simulink model "ARC_DTm"  (R2025b)
settings: Solver=FixedStepAuto  StartTime=0.0  StopTime=10080  FixedStep=1  RelTol=1e-3
PreLoadFcn:
  | %For Preload, set the working path
  | modelFolder = fileparts(which(bdroot));
  | addpath(genpath(modelFolder));
StartFcn:
  | tic
StopFcn:
  | fprintf("Sim Time: %.02f min", toc/60)
values from neighbouring files (symbols this model uses):
  batteryScenario = p.batteryScenario    [RUNSIM_ParameterSweep.m]    (also in _RUNSIM_ParameterSweep.m)
  Electricity_SalePriceModifier = 50/100    (= 0.5)    [RUNSIM_ParameterSweep.m]    (also in _RUNSIM_ParameterSweep.m)
  LUT = LUT_load.gamLUT    [RUNSIM_ParameterSweep.m]    (also in _RUNSIM_ParameterSweep.m)
  minimum_UF_system_flow = 5833    [RUNSIM_ParameterSweep.m]    (also in _RUNSIM_ParameterSweep.m)
  PROS1_recoveryrate = 61    [RUNSIM_ParameterSweep.m]    (also in _RUNSIM_ParameterSweep.m)
  PROS2_recoveryrate = 62    [RUNSIM_ParameterSweep.m]    (also in _RUNSIM_ParameterSweep.m)
  ROstabilization_time = p.ROstabilization_time    [RUNSIM_ParameterSweep.m]    (also in _RUNSIM_ParameterSweep.m)
  solarModifier = maximum_solar_generation / 300    [RUNSIM_ParameterSweep.m]    (also in _RUNSIM_ParameterSweep.m)
  TSRO_recoveryrate = 51    [RUNSIM_ParameterSweep.m]    (also in _RUNSIM_ParameterSweep.m)
  UF_RecoveryRate = 96    [RUNSIM_ParameterSweep.m]    (also in _RUNSIM_ParameterSweep.m)
undefined symbols (not defined in the file or in its folder): A_PROS1, A_PROS2, A_TSRO, B_PROS1, B_PROS2, B_TSRO, BW_Max_Time, BW_Max_Vol_gal, CEB_Max_Time, CEB_Max_Vol_gal, CIP_Max_Time, E, FF, h, L, w
libraries: simulink x40
(part 3 of 11)

== system ARC_DTm/Plant_LocalLoad_FMU ==
  note: Time-of-Use Scenarios are defined in the input spreadsheet 'OperationalScenarios.xlsx'. This subsystem allows a toggling of scenarios through modifying the TOU_Rate_Scenario constant block in the MATLAB editor.
  note: Net Power
  note: PRO_1
  note: Import UF Power
  note: PRO_2
  note: PRO_3
  note: PRO_4
  note: This subsystem utilizes the FMU and battery logic developed by the Electric Power Research Institute (EPRI) to simulate the potential impact of an on-site battery under different charge and discharge control scenarios.
  Abs : Abs  SaturateOnIntegerOverflow=off
  Abs1 : Abs  SaturateOnIntegerOverflow=off
  Add : Sum
  Add1 : Sum  Inputs=++++
  Add2 : Sum  Inputs=++++++++
  Add3 : Sum  Inputs=++++
  Battery System : Subsystem
  Bus Creator : BusCreator  Inputs=27
  Constant : Constant  Value=0
  Decarb Off : Constant  Value=0
  Decarbonator Power Demand_kW : Constant  Value=2.5
  Demux : Demux
  Energy Summary : Scope  NumInputPorts=4
      settings: ActiveDisplayYMinimum=-0.12499999999999997  ActiveDisplayYMaximum=1.125  DataLoggingVariableName=ScopeData20
  FMU : FMU  FMUName=HybridPowerControls_EPRI.fmu  FMUDebugLogging=on  FMUMode=CoSimulation  FMUInitializeEnumObject=off  FMUCachedDialogLayout="{\"Geometry\":[0,186,578,484],\"ParameterColumnsWidthConfig\":\"{\\\"columns\\\":[{\\\"name\\\":\\\"Parameter\\\",\\\"width\\\":154},{\\\"name\\\":\\\"Value\\\",\\\"width\\\":59},{\\\"name\\\":\\\"Calculated Value\\\",\\\"width\\\":203},{\\\"name\\\":\\\"Unit\\\",\\\"width\\\":108},{\\\"name\\\":\\\"Description\\\",\\\"width\\\":161}]}\",\"InputColumnsWidthConfig\":\"{\\\"columns\\\":[{\\\"name\\\":\\\"Name\\\",\\\"width\\\":150},{\\\"name\\\":\\\"Visibility\\\",\\\"width\\\":79},{\\\"name\\\":\\\"Start\\\",\\\"width\\\":139},{\\\"name\\\":\\\"Unit\\\",\\\"width\\\":136},{\\\"name\\\":\\\"Type Object\\\",\\\"width\\\":194}]}\",\"OutputColumnsWidthConfig\":\"{\\\"columns\\\":[{\\\"name\\\":\\\"Name\\\",\\\"width\\\":150},{\\\"name\\\":\\\"Visibility\\\",\\\"width\\\":79},{\\\"name\\\":\\\"Start\\\",\\\"width\\\":139},{\\\"name\\\":\\\"Unit\\\",\\\"width\\\":136},{\\\"name\\\":\\\"Type Object\\\",\\\"width\\\":194}]}\"}"  DCDC=struct('P_rat',0,'P_ref',5.0E7,'V_ref',1.0,'capex_ref',1.0,'componentEconomy',struct('annualCapex',0,'capex',0,'cashFlowPerSecond',0,'fixedAnnualOpex',0,'lifetime',0,'summary',struct('capex',0)),'constraint_prim',struct('upperLimitFixed',1.0),'constraint_sec',struct('lowerLimitFixed',-1.0,'upperLimitFixed',1.0),'eta',1.0,'fixedAnnualOpex_ref',1.0,'lifetime',1.0,'pin_prim',struct('v',0),'pin_sec',struct('v',0),'scalingFactor',1.0,'scalingFactor_max',10.0,'scalingFactor_min',0.1,'smoothingPercentage',2.0)  PID_charge=struct('Dzero',struct('k',0.0,'y',0),'FFzero',struct('k',0.0,'y',0),'I',struct('k',0,'y_start',0),'Nd',10.0,'Ni',0.9,'P',struct('k',1.0),'Td',0.1,'Ti',0.025,'addFF',struct('k1',1.0,'k2',0,'u2',0),'addI',struct('k1',1.0,'k2',-1.0,'k3',1.0),'addP',struct('k1',0,'k2',-1.0),'addPID',struct('k1',1.0,'k2',1.0,'k3',1.0,'u2',0),'addSat',struct('k1',1.0,'k2',-1.0),'gainPID',struct('k',0),'gainTrack',struct('k',0),'k',0.16,'kFF',1.0,'wd',0.0,'wp',1.0,'xd_start',0.0,'xi_start',0.0)  PID_discharge=struct('Dzero',struct('k',0.0,'y',0),'FFzero',struct('k',0.0,'y',0),'I',struct('k',0,'y_start',0),'Nd',10.0,'Ni',0.9,'P',struct('k',1.0),'Td',0.1,'Ti',0.025,'addFF',struct('k1',1.0,'k2',0,'u2',0),'addI',struct('k1',1.0,'k2',-1.0,'k3',1.0),'addP',struct('k1',0,'k2',-1.0),'addPID',struct('k1',1.0,'k2',1.0,'k3',1.0,'u2',0),'addSat',struct('k1',1.0,'k2',-1.0),'gainPID',struct('k',0),'gainTrack',struct('k',0),'k',0.16,'kFF',1.0,'wd',0.0,'wp',1.0,'xd_start',0.0,'xi_start',0.0)  P_block_jacobian_check=off  P_block_jacobian_check_tol=1.0E-6  P_block_solver_experimental_mode=int32(0)  P_block_solver_profiling=off  P_cs_experimental_mode=int32(0)  P_cs_profiling=off  P_cs_rel_tol=1.0E-6  P_cs_solver=int32(0)  P_cs_step_size=0.001  P_enforce_bounds=on  P_events_default_tol=1.0E-10  P_events_tol_factor=1.0E-4  P_iteration_variable_scaling=int32(1)  P_log_level=int32(3)  P_log_start_time=-1.0E20  P_log_stop_time=1.0E20  P_mathematical_domain_warnings_limit=int32(-1)  P_nle_active_bounds_mode=int32(0)  P_nle_brent_ignore_error=off  P_nle_jacobian_calculation_mode=int32(0)  P_nle_jacobian_finite_difference_delta=1.490116119384766E-8  P_nle_jacobian_update_mode=int32(2)  P_nle_solver_check_jac_cond=off  P_nle_solver_default_tol=1.0E-10  P_nle_solver_exit_criterion=int32(3)  P_nle_solver_max_iter=int32(100)  P_nle_solver_max_iter_no_jacobian=int32(10)  P_nle_solver_max_residual_scaling_factor=1.0E10  P_nle_solver_min_residual_scaling_factor=1.0E-10  P_nle_solver_min_tol=1.0E-12  P_nle_solver_regularization_tolerance=-1.0  P_nle_solver_step_limit_factor=10.0  P_nle_solver_tol_factor=1.0E-4  P_nle_solver_use_last_integrator_step=on  P_nle_solver_use_nominals_as_fallback=on  P_rescale_after_singular_jac=on  P_rescale_each_step=off  P_residual_equation_scaling=int32(1)  P_runtime_log_to_file=off  P_time_events_default_tol=2.220446049250313E-14  P_time_events_min_tol=2.220446049250313E-14  P_use_Brent_in_1d=on  P_use_jacobian_equilibration=off  P_use_newton_for_brent=on  battery=struct('P_el_max',0,'SOC_max',0.95,'SOC_min',0.05,'SOC_start',0.15,'capacity_rat',0,'capacity_ref',1.4399999999999988E11,'capex_ref',9000000.0,'componentEconomy',struct('annualCapex',0,'capex',0,'cashFlowPerSecond',0,'fixedAnnualOpex',0,'lifetime',0,'summary',struct('capex',0)),'constraint_P_el',struct('lowerLimitFixed',0,'upperLimitFixed',0),'constraint_SOC',struct('lowerLimitFixed',0,'upperLimitFixed',0),'eta_charge',0.95,'eta_discharge',0,'fixedAnnualOpex_ref',0,'lifetime',10.0,'pin_DC',struct('v',0),'scalingFactor',1.0,'scalingFactor_max',10.0,'scalingFactor_min',0.1,'set_SOC_final_start_',boolean(false))  boundary_AC=struct('E_el_max',0.0,'E_el_min',0.0,'P_el_max',1.0E60,'V_port',0,'V_ref',1.0,'constraint_E_el',struct('lowerLimitFixed',0,'t_constraint',0,'targetValue',0.0,'upperLimitFixed',0,'useTargetValue',boolean(false)),'constraint_V',struct('constraintTarget',0,'lowerLimitFixed',0,'upperLimitFixed',0),'pin_AC',struct('v',[0]))  boundary_AC2=struct('E_el_max',0.0,'E_el_min',0.0,'P_el_max',1.0E60,'V_port',0,'V_ref',1.0,'constraint_E_el',struct('lowerLimitFixed',0,'t_constraint',0,'targetValue',0.0,'upperLimitFixed',0,'useTargetValue',boolean(false)),'constraint_P_el',struct('lowerLimitFixed',0.0,'upperLimitFixed',0),'flowDirection',int32(1),'pin_AC',struct('v',[0]))  economy=struct('annualCapex',0,'capex',0,'capex_max',1.0E60,'disableSimTimeWarning',boolean(false),'economyConnector',struct('annualCapex',0,'capex',0,'fixedAnnualOpex',0),'fixedAnnualOpex',0,'objectiveIntegrands',struct('capex',0),'summary',struct('capex',0))  electricityPurchase=struct('E_el_max',0.0,'E_el_min',0.0,'P_el_max',1.0E60,'V_port',0,'V_ref',1.0,'componentEconomy',struct('annualCapex',0,'capex',0.0,'fixedAnnualOpex',0.0,'lifetime',1.0,'summary',struct('capex',0)),'constraint_E_el',struct('lowerLimitFixed',0,'t_constraint',0,'targetValue',0.0,'upperLimitFixed',0,'useTargetValue',boolean(false)),'constraint_V',struct('constraintTarget',0,'lowerLimitFixed',0.0,'upperLimitFixed',0),'pin_AC',struct('v',[0]))  electricitySale=struct('E_el_max',0.0,'E_el_min',0.0,'P_el_max',1.0E60,'V_port',0,'V_ref',1.0,'componentEconomy',struct('annualCapex',0,'capex',0.0,'fixedAnnualOpex',0.0,'lifetime',1.0,'summary',struct('capex',0)),'constraint_E_el',struct('lowerLimitFixed',0,'t_constraint',0,'targetValue',0.0,'upperLimitFixed',0,'useTargetValue',boolean(false)),'constraint_V',struct('constraintTarget',0,'lowerLimitFixed',0,'upperLimitFixed',0),'pin_AC',struct('v',[0]))  gain=struct('k',-1.0)  gain2=struct('k',0)  gain4=struct('k',0)  hysteresis_max=struct('pre_y_start',boolean(false),'uHigh',0,'uLow',0)  hysteresis_min=struct('pre_y_start',boolean(false),'uHigh',0,'uLow',0)  inverter=struct('P_rat',0,'P_ref',1.5E8,'V_ref',1.0,'capex_ref',1.0,'componentEconomy',struct('annualCapex',0,'capex',0,'cashFlowPerSecond',0,'fixedAnnualOpex',0,'lifetime',0,'summary',struct('capex',0)),'constraint_prim',struct('upperLimitFixed',1.0),'eta',0.99,'fixedAnnualOpex_ref',1.0,'lifetime',1.0,'pin_prim',struct('v',0),'pin_sec',struct('v',[0]),'scalingFactor',1.0,'scalingFactor_max',10.0,'scalingFactor_min',0.1,'smoothingPercentage',2.0)  optimizer=struct('filterHiddenResults',boolean(true),'includeSimResult',boolean(false),'ipoptMaxIterations',int32(3000),'ipoptTolerance',1.0E-8,'linearSolver',int32(1),'ma57PivotTolerance',1.0E-8,'n_blockedElements',int32(1),'n_collocationPoints',int32(1),'quadraticPenalty',0.0,'samplingTime',3600.0,'t_opt_end',86400.0,'t_opt_start',0.0,'t_preSimulation_start',0.0,'useBlockingFactors',boolean(true),'useElimination',boolean(true),'useQuadraticPenalty',boolean(false))  photovoltaics=struct('P_el_rat',0,'P_el_ref',1.0,'capex_ref',400.0,'componentEconomy',struct('annualCapex',0,'capex',0,'cashFlowPerSecond',0,'fixedAnnualOpex',0,'lifetime',0,'summary',struct('capex',0)),'fixedAnnualOpex_ref',10.0,'lifetime',25.0,'pin_DC',struct('v',0),'scalingFactor',1.0,'scalingFactor_max',10.0,'scalingFactor_min',0.1)  pulse=struct('amplitude',8500000.0,'nperiod',int32(-1),'offset',0.0,'period',86400.0,'startTime',25200.0,'width',41.66)  transferFunction=struct('a',[300.0,1.0],'b',[1.0],'x_start',[0.0],'y_start',0.0)  trapezoid=struct('amplitude',8500000.0,'falling',5400.0,'nperiod',int32(-1),'offset',0.0,'period',43200.0,'rising',5400.0,'startTime',19800.0,'width',10800.0)  unitDelay=struct('samplePeriod',0.1,'startTime',0.0,'y_start',0.0)  unitDelay2=struct('samplePeriod',0.1,'startTime',0.0,'y_start',0.0)  mask(hybrid_power_controls.hp_bat_3_FMU_NAWI [Co-Simulation, v2.0]){}
      mask Display:
      | disp('hybrid_power_controls.hp_bat_3_FMU_NAWI');
      | port_label('output',1,'Batt_Pel');
      | port_label('output',2,'Batt_Pgross');
      | port_label('output',3,'Batt_SOC');
      | port_label('output',4,'Boundary_AC2_Pel');
      | port_label('output',5,'Electr_Purchase_Pel');
      | port_label('output',6,'Electr_Sale_Pel');
      | port_label('output',7,'Var_Opex_per_sec');
      | port_label('input',1,'Batt_Charge');
      | port_label('input',2,'Batt_Discharge');
      | port_label('input',3,'LocalLoadDemand_kW');
      | port_label('input',4,'PurchasePower_Dollar_per_kWh');
      | port_label('input',5,'PurchasePower_W');
      | port_label('input',6,'SalePower_Dollar_per_kWh');
      | port_label('input',7,'SalePower_W');
      | port_label('input',8,'Solar_in_kW');
  Gain : Gain  Gain=Electricity_SalePriceModifier
  Gain1 : Gain  Gain=1/1000
  Integrator : Integrator
  Max : MinMax  Function=max  Inputs=2
  Memory : Memory
  Min : MinMax  Inputs=2
  Minus : Sum  Inputs=+-
  NetPower : Scope  NumInputPorts=4
      settings: ActiveDisplayYMinimum=-1907.3777939419972  ActiveDisplayYMaximum=1672.6343144261821  DataLoggingVariableName=ScopeData36
  Plant_SolarGeneration : Scope  NumInputPorts=2
      settings: ActiveDisplayYMinimum=-156.91113785545454  ActiveDisplayYMaximum=1412.2002406990912  DataLoggingVariableName=ScopeData45
  Product : Product
  Product1 : Product
  Scope : Scope  NumInputPorts=7
      settings: ActiveDisplayString=5  ActiveDisplayYMinimum=-123823.38700118322  ActiveDisplayYMaximum=1.1144104830106492E+6  DataLoggingVariableName=ScopeData50
  Scope1 : Scope  NumInputPorts=6
      settings: ActiveDisplayYMinimum=-1  ActiveDisplayYMaximum=1  DataLoggingVariableName=ScopeData25
  Scope2 : Scope  NumInputPorts=8
      settings: ActiveDisplayYMinimum=-50.191836395021646  ActiveDisplayYMaximum=451.72652755519493  DataLoggingVariableName=ScopeData46
  Scope5 : Scope
      settings: ActiveDisplayYMinimum=-26.16015827516069  ActiveDisplayYMaximum=235.44142447644629  DataLoggingVariableName=ScopeData30
  Sum : Sum
  Sum1 : Sum
  Sum2 : Sum
  Sum3 : Sum  Inputs=|++
  Sum4 : Sum  Inputs=+-+
  Switch : Switch  Criteria=u2 > Threshold  SaturateOnIntegerOverflow=off  InputSameDT=off
  Switch1 : Switch  Criteria=u2 > Threshold  SaturateOnIntegerOverflow=off  InputSameDT=off
  To Workspace : ToWorkspace  VariableName=power  SaveFormat=Timeseries  SampleTime=-1
  Total Energy Costs : Integrator
  kW>MW : Gain  Gain=1/1000
  wires:
  Abs/1 -> kW>MW/1
  [UF_PumpPower_Vector] -> Scope5/1, Demux/1
  Demux/1 -> Bus Creator/1, Add1/1  "UFPump_1_Power"
  Demux/2 -> Bus Creator/2, Add1/2  "UFPump_2_Power"
  Demux/3 -> Add1/4, Bus Creator/4  "UFPump_3_Power"
  Demux/4 -> Add1/3, Bus Creator/3  "UFPump_4_Power"
  [PROS1_1_Power_kW] -> Bus Creator/5, Sum/1  "PROS1_1_Power_kW"
  [PROS2_1_Power_kW] -> Bus Creator/6, Sum/2  "PROS2_1_Power_kW"
  [PROS1_2_Power_kW] -> Bus Creator/7, Sum1/1  "PROS1_2_Power_kW"
  [PROS2_2_Power_kW] -> Bus Creator/8, Sum1/2  "PROS2_2_Power_kW"
  [PROS1_3_Power_kW] -> Bus Creator/9, Sum2/1  "PROS1_3_Power_kW"
  [PROS2_3_Power_kW] -> Bus Creator/10, Sum2/2  "PROS2_3_Power_kW"
  [PROS2_4_Power_kW] -> Bus Creator/11, Add/1  "PROS1_4_Power_kW"
  [PROS2_4_Power_kW] -> Bus Creator/12, Add/2  "PROS2_4_Power_kW"
  Sum/1 -> Scope2/2, Add2/2  "PRO1_NetPowerDemand"
  [UVAOP_1_kW] -> Bus Creator/17, Sum3/1  "UVAOP_1_Power_kW"
  [UVAOP_2_kW] -> Bus Creator/18, Sum3/2  "UVAOP_2_Power_kW"
  Add1/1 -> Scope2/1, Add2/1  "UF_NetPowerDemand"
  Sum1/1 -> Scope2/3, Add2/3  "PRO2_NetPowerDemand"
  Sum2/1 -> Add2/4, Scope2/4  "PRO3_NetPowerDemand"
  Add/1 -> Add2/5, Scope2/5  "PRO4_NetPowerDemand"
  [TSRO_1_Power_kW] -> Bus Creator/13, Add3/1  "TSRO_1_Power_kW"
  [TSRO_2_Power_kW] -> Bus Creator/14, Add3/2  "TSRO_2_Power_kW"
  [TSRO_3_Power_kW] -> Bus Creator/15, Add3/3  "TSRO_3_Power_kW"
  [TSRO_4_Power_kW] -> Bus Creator/16, Add3/4  "TSRO_4_Power_kW"
  Add3/1 -> Scope2/6, Add2/6
  Sum3/1 -> Add2/7, Scope2/7, Switch/2  "UVAOP_NetPowerDemand"
  Decarbonator Power Demand_kW/1 -> Switch/1
  Decarb Off/1 -> Switch/3
  Switch/1 -> Scope2/8, Add2/8, Bus Creator/19  "Decarbonator_Power_kW"
  Add2/1 -> Sum4/1, NetPower/1, Bus Creator/20, Battery System/2(Local Load Demand), Minus/2, Scope1/1, FMU/3, Plant_SolarGeneration/1  "Plant_LocalPowerDemand_kW"
  [Plant_SolarPower_kW] -> Plant_SolarGeneration/2, NetPower/2, Sum4/2, Bus Creator/25, Minus/1, Abs/1, Battery System/1(Solar In)  "Plant_SolarGeneration_kW"
  Bus Creator/1 -> To Workspace/1
  Sum4/1 -> Product1/2, Switch1/2, Product/1, Bus Creator/21, NetPower/4, Integrator/1  "Plant_NetPowerDemand_kW"
  Gain/1 -> Bus Creator/22, Product1/1, FMU/6, Scope1/4  "Plant_ Electricity_SalePrice_dol_kWh"
  FMU/2 -> Scope/2  "Batt_Pgross"
  FMU/1 -> Gain1/1  "Plant_Battery_Power_kW"
  FMU/3 -> Battery System/3(SOC), Scope/3  "Batt_SOC"
  FMU/4 -> Energy Summary/4, Memory/1, Scope/4  "Boundary_AC2_Pel"
  FMU/5 -> Scope/5  "Electr_Purchase_Pel"
  kW>MW/1 -> Scope1/6, FMU/8  "Solar in _MW"
  Constant/1 -> Max/2, Min/2
  Max/1 -> Scope1/5, FMU/7  "SalePower_W"
  Memory/1 -> Min/1, Max/1
  Min/1 -> Abs1/1
  Abs1/1 -> Scope1/3, FMU/5
  Integrator/1 -> Bus Creator/23  "Plant_TotalPowerDemand_kWh"
  [TOURates] -> Product/2, Bus Creator/24, FMU/4, Scope1/2, Gain/1  "Plant_TOURate"
  Battery System/1(Battery Charge) -> Energy Summary/1, FMU/1  "Charge Command"
  Battery System/2(Battery  discharge) -> Energy Summary/2, FMU/2  "Discharge Command"
  Minus/1 -> Energy Summary/3  "Net Power Demand"
  FMU/6 -> Scope/6  "Electr_Sale_Pel"
  FMU/7 -> Scope/7  "Var_Opex_per_sec"
  Product/1 -> Switch1/1
  Total Energy Costs/1 -> Bus Creator/27  "Plant_TotalEnergyCosts_dol"
  Switch1/1 -> Total Energy Costs/1
  Product1/1 -> Switch1/3
  Gain1/1 -> Bus Creator/26, NetPower/3, Sum4/3, Scope/1  "Plant_Battery_Power_kW"

== system ARC_DTm/Process Constants ==
  note: Reverse Osmosis Membrane Constants
      | This section is largely defined in the initialization script as seen in the 'InitFcn' under Modeling > Model Properties > Model Callbacks.
      | Element and vessel data is found in plant design documentation. Spacer Porosity was found using WaterTAP parameter estimation. Water and salt permeability values were found using MATLAB's Parameter Estimation app through signal matching with
      | operational data.
  Bus Creator : BusCreator  Inputs=3
  Bus Creator1 : BusCreator  Inputs=3
  Bus Creator2 : BusCreator  Inputs=3
  Bus Creator3 : BusCreator  Inputs=2
  Bus Creator4 : BusCreator  Inputs=2
  Filtrate Pressure MAX (psi) : Constant  Value=39
  Filtrate Pressure Ratio (dmnl) : Constant  Value=.89
  Membrane Area (ft^2) : Constant  Value=775
  Membranes per Skid : Constant  Value=80
  PROS1_MembraneArea_m2 : Product
  PROS1_VesselsperSkid : Constant  Value=72
  PROS2_MembraneArea_m : Product
  PROS2_Suction_PressureDrop_psi : Constant  Value=7
  PROS2_VesselsperSkid : Constant  Value=40
  PROStage1_SaltPermeability_m3_m2s : Constant  Value=B_PROS1
  PROStage1_WaterPermeability_m3_m2spsi : Constant  Value=A_PROS1*1.18
  PROStage2_SaltPermeability_m3_m2s : Constant  Value=B_PROS2
  PROStage2_WaterPermeability_m3_m2spsi : Constant  Value=A_PROS2
  RO_AreaperVessel_m2 : Product  Inputs=3
  RO_ElementArea_ft2 : Constant  Value=400
  RO_ElementsperVessel : Constant  Value=7
  RO_PermeatePressure_psi : Constant  Value=20
  RO_SpacerPorosity : Constant  Value=E
  TSRO_MembraneArea_m : Product
  TSRO_SaltPermeability_m3_m2s : Constant  Value=B_TSRO
  TSRO_Suction_PressureDrop_psi : Constant  Value=60
  TSRO_VesselsperSkid : Constant  Value=30
  TSRO_WaterPermeability_m3_m2spsi : Constant  Value=A_TSRO*.55
  Total Membrane Area (ft^2) : Product
  UF_Pump_MaxFlow_gpm : Constant  Value=3850
  UF_Pump_MinFlow_gpm : Constant  Value=918
  cm2>m2 : Gain  Gain=1/10000
  ft2>in2 : Gain  Gain=144
  in2>cm2 : Gain  Gain=2.54^2
  uScm_to_mg/L_TDS : Constant  Value=.5
  tag scope: PROS1_MembraneConstants=global, PROS2_MembraneConstants=global, PROS2_Suction_PressureDrop_psi=global, RO_PermeatePressure=global, TSRO_MembraneConstants=global, TSRO_Suction_PressureDrop_psi=global, UFPump_Bounds=global, UF_MaxFiltratePressure=global, UF_MembraneCharacteristics=global, sal=global
  wires:
  RO_ElementArea_ft2/1 -> ft2>in2/1
  TSRO_VesselsperSkid/1 -> TSRO_MembraneArea_m/1
  PROStage1_SaltPermeability_m3_m2s/1 -> Bus Creator/2  "PROS1_B"
  ft2>in2/1 -> in2>cm2/1
  RO_ElementsperVessel/1 -> RO_AreaperVessel_m2/3
  RO_SpacerPorosity/1 -> RO_AreaperVessel_m2/1
  in2>cm2/1 -> cm2>m2/1
  PROS1_VesselsperSkid/1 -> PROS1_MembraneArea_m2/1
  cm2>m2/1 -> RO_AreaperVessel_m2/2
  RO_AreaperVessel_m2/1 -> TSRO_MembraneArea_m/2, PROS2_MembraneArea_m/2, PROS1_MembraneArea_m2/2
  TSRO_SaltPermeability_m3_m2s/1 -> Bus Creator2/2  "TSRO_B"
  PROS2_VesselsperSkid/1 -> PROS2_MembraneArea_m/1
  PROStage1_WaterPermeability_m3_m2spsi/1 -> Bus Creator/1  "PROS1_A"
  PROS1_MembraneArea_m2/1 -> Bus Creator/3  "PROS1_Area_m2"
  TSRO_WaterPermeability_m3_m2spsi/1 -> Bus Creator2/1  "TSRO_A"
  TSRO_MembraneArea_m/1 -> Bus Creator2/3  "TSRO_Area_m2"
  PROStage2_WaterPermeability_m3_m2spsi/1 -> Bus Creator1/1  "PROS2_A"
  PROStage2_SaltPermeability_m3_m2s/1 -> Bus Creator1/2  "PROS2_B"
  PROS2_MembraneArea_m/1 -> Bus Creator1/3  "PROS2_Area_m2"
  Bus Creator/1 -> [PROS1_MembraneConstants]
  Bus Creator2/1 -> [TSRO_MembraneConstants]
  Bus Creator1/1 -> [PROS2_MembraneConstants]
  RO_PermeatePressure_psi/1 -> [RO_PermeatePressure]
  uScm_to_mg/L_TDS/1 -> [sal]
  Membranes per Skid/1 -> Total Membrane Area (ft^2)/2
  Total Membrane Area (ft^2)/1 -> [UF_MembraneCharacteristics]  "Membrane Area (ft^2)"
  Membrane Area (ft^2)/1 -> Total Membrane Area (ft^2)/1
  Filtrate Pressure MAX (psi)/1 -> Bus Creator3/1  "UF_MaxFiltratePressure_psi"
  Filtrate Pressure Ratio (dmnl)/1 -> Bus Creator3/2  "UF_FiltratePressureRatio"
  Bus Creator3/1 -> [UF_MaxFiltratePressure]
  PROS2_Suction_PressureDrop_psi/1 -> [PROS2_Suction_PressureDrop_psi]
  TSRO_Suction_PressureDrop_psi/1 -> [TSRO_Suction_PressureDrop_psi]
  UF_Pump_MaxFlow_gpm/1 -> Bus Creator4/1  "MaxFlow_gpm"
  UF_Pump_MinFlow_gpm/1 -> Bus Creator4/2  "MinFlow_gpm"
  Bus Creator4/1 -> [UFPump_Bounds]

== system ARC_DTm/Product Water Tank ==
  note: V(t) dc/dt = W(t) - c(t)[Vset * As + k * V(t) + Qout(t)]
      | dc / dt = [W(t) - c(t)[Qout(t)]]/V(t)
      | dV/dt = Qin - Qout
      | find minimum operating volume
  Raw Water Inflow : Inport
  RO Permeate Flow : Inport  Port=2
  Pump Flow : Inport  Port=3
  Bus Creator : BusCreator  Inputs=3
  Bus Creator1 : BusCreator  Inputs=2
  Bus Selector : BusSelector  OutputSignals=Temp (*C),TSS (CONC),Salinity (CONC),RequestedFlow (FLOW)
  Bus Selector1 : BusSelector  OutputSignals=Permeate Flow (FLOW),Temperature (*C),TSD (CONC),TSS (CONC)
  Bus to Vector : BusToVector
  Constant : Constant  Value=vol
  Gain : Gain  Gain=volMax
  Gain1 : Gain  Gain=volMin
  Inflow 1 Flow Rate (FLOW) : Selector  InputPortWidth=2  IndexOptions=Starting index (dialog)  Indices=[1]  OutputSizes=1
  Inflow 2 Flow Rate (FLOW) : Selector  InputPortWidth=2  IndexOptions=Index vector (dialog)  Indices=2  OutputSizes=1
  Integrator : Integrator  InitialCondition=initVol * vol
  MATLAB Function : MATLAB Function  TreatAsAtomicUnit=on
  Memory : Memory  LinearizeAsDelay=on
  Permeate TSS Loading Rate : Product
  Permeate Temperature Loading Rate : Product
  Product : Product
  Product1 : Product
  RW Loading Rate : Product
  RW Temp Loading Rate (*C/s) : Product
  Salinity Mass Balance : Subsystem
      settings: PortSchema="{\"entries\":[{\"content\":{\"sides\":[{\"content\":{\"connectorIds\":[\"In1\",\"In2\"]},\"type\":\"ConnectorPlacement.EquallySpacedRectSide\",\"uuid\":\"dcb8863d-ddb0-40a4-b080-865306d6a008\"},{\"content\":{\"connectorIds\":[\"Out1\"],\"side\":\"RIGHT\"},\"type\":\"ConnectorPlacement.EquallySpacedRectSide\",\"uuid\":\"89be541c-ebd4-4185-8b67-61e08e91f446\"},{\"content\":{\"side\":\"TOP\"},\"type\":\"ConnectorPlacement.EquallySpacedRectSide\",\"uuid\":\"09d290c4-cbf6-44b9-a242-0cdebe116f52\"},{\"content\":{\"connectorIds\":[\"In3\",\"In4\",\"In5\"],\"side\":\"BOTTOM\"},\"type\":\"ConnectorPlacement.EquallySpacedRectSide\",\"uuid\":\"3fed9ad6-9e0e-418c-9a39-4247b7dc8415\"}]},\"type\":\"ConnectorPlacement.EquallySpacedConnector\",\"uuid\":\"c64f9444-fa85-4c04-9a4b-bca16ff2b046\"}],\"packageUris\":[\"http://schema.mathworks.com/mf0/Connector/R2020b\"],\"version\":\"1.0\"}"
  Scope : Scope  NumInputPorts=3
      settings: ActiveDisplayYMinimum=253.84635834993  ActiveDisplayYMaximum=253.84635835033
  Scope1 : Scope  NumInputPorts=3
      settings: ActiveDisplayYMinimum=10.10463  ActiveDisplayYMaximum=46.65504
  Scope2 : Scope  NumInputPorts=2
      settings: ActiveDisplayYMinimum=-1.75  ActiveDisplayYMaximum=15.75
  Scope3 : Scope  NumInputPorts=2
      settings: ActiveDisplayYMinimum=-6.25  ActiveDisplayYMaximum=56.25  DataLoggingVariableName=ScopeData2
  TSS Mass Balance : Subsystem
      settings: PortSchema="{\"entries\":[{\"content\":{\"sides\":[{\"content\":{\"connectorIds\":[\"In1\",\"In2\"]},\"type\":\"ConnectorPlacement.EquallySpacedRectSide\",\"uuid\":\"dcb8863d-ddb0-40a4-b080-865306d6a008\"},{\"content\":{\"connectorIds\":[\"Out1\"],\"side\":\"RIGHT\"},\"type\":\"ConnectorPlacement.EquallySpacedRectSide\",\"uuid\":\"89be541c-ebd4-4185-8b67-61e08e91f446\"},{\"content\":{\"side\":\"TOP\"},\"type\":\"ConnectorPlacement.EquallySpacedRectSide\",\"uuid\":\"09d290c4-cbf6-44b9-a242-0cdebe116f52\"},{\"content\":{\"connectorIds\":[\"In3\",\"In4\",\"In5\"],\"side\":\"BOTTOM\"},\"type\":\"ConnectorPlacement.EquallySpacedRectSide\",\"uuid\":\"3fed9ad6-9e0e-418c-9a39-4247b7dc8415\"}]},\"type\":\"ConnectorPlacement.EquallySpacedConnector\",\"uuid\":\"c64f9444-fa85-4c04-9a4b-bca16ff2b046\"}],\"packageUris\":[\"http://schema.mathworks.com/mf0/Connector/R2020b\"],\"version\":\"1.0\"}"
  Tank Storage : Subsystem  Commented=on
  Temperature Balance : Subsystem
      settings: PortSchema="{\"entries\":[{\"content\":{\"sides\":[{\"content\":{\"connectorIds\":[\"In1\",\"In2\"]},\"type\":\"ConnectorPlacement.EquallySpacedRectSide\",\"uuid\":\"9127f392-a9e0-4f8f-80b5-81b1619eb257\"},{\"content\":{\"connectorIds\":[\"Out1\"],\"side\":\"RIGHT\"},\"type\":\"ConnectorPlacement.EquallySpacedRectSide\",\"uuid\":\"c9fcd324-2499-4af3-8e50-54b134b6fd5a\"},{\"content\":{\"side\":\"TOP\"},\"type\":\"ConnectorPlacement.EquallySpacedRectSide\",\"uuid\":\"ae0b57ef-93cf-4f11-b6be-33f2d8da1cc8\"},{\"content\":{\"connectorIds\":[\"In3\",\"In4\",\"In5\"],\"side\":\"BOTTOM\"},\"type\":\"ConnectorPlacement.EquallySpacedRectSide\",\"uuid\":\"9c672c45-ba7a-4af9-a87c-581d143eff6a\"}]},\"type\":\"ConnectorPlacement.EquallySpacedConnector\",\"uuid\":\"ebc50df8-8afe-413b-baf9-e0176f22e6f7\"}],\"packageUris\":[\"http://schema.mathworks.com/mf0/Connector/R2020b\"],\"version\":\"1.0\"}"
  Out1 : Outport
  ActualOutflow1 (FLOW) : Outport  Port=2
  ActualInflow1 (FLOW) : Outport  Port=3
  ActualInflow2 (FLOW) : Outport  Port=4
  wires:
  Raw Water Inflow/1 -> Bus Selector/1
  Bus Selector/2 -> RW Loading Rate/1  "<TSS (CONC)>"
  RW Loading Rate/1 -> TSS Mass Balance/1(InflowLoadingRate1)  "LOADING"
  Bus Creator/1 -> Out1/1  "RawWaterQualityCharacteristics"
  Bus Selector/1 -> RW Temp Loading Rate (*C/s)/1  "<Temp (*C)>"
  RO Permeate Flow/1 -> Bus Selector1/1
  Bus Selector1/2 -> Permeate Temperature Loading Rate/1  "<Temperature (*C)>"
  Bus Selector1/4 -> Permeate TSS Loading Rate/2  "<TSS (CONC)>"
  Permeate TSS Loading Rate/1 -> TSS Mass Balance/2(InflowLoadingRate2)  "LOADING"
  Bus Selector1/1 -> Bus Creator1/2  "<Permeate Flow (FLOW)>"
  Inflow 1 Flow Rate (FLOW)/1 -> Product/2, RW Loading Rate/2, RW Temp Loading Rate (*C/s)/2, ActualInflow1 (FLOW)/1  "Well Flow Rate (FLOW)"
  Inflow 2 Flow Rate (FLOW)/1 -> ActualInflow2 (FLOW)/1, Permeate Temperature Loading Rate/2, Product1/1, Permeate TSS Loading Rate/1  "RO Perm Flow Rate (FLOW)"
  MATLAB Function/2(newOutflows) -> ActualOutflow1 (FLOW)/1, TSS Mass Balance/3(OutflowRate1), Temperature Balance/3(OutflowRate1 (flow)), Salinity Mass Balance/3(OutflowRate1), Scope3/2  "Pump Flow Rate (FLOW)"
  Pump Flow/1 -> MATLAB Function/2(outflows)
  Bus Selector/4 -> Bus Creator1/1  "<RequestedFlow (FLOW)>"
  Permeate Temperature Loading Rate/1 -> Temperature Balance/2(InflowLoadingRate2)
  RW Temp Loading Rate (*C/s)/1 -> Temperature Balance/1(InflowLoadingRate1)
  MATLAB Function/3(dVdt) -> Integrator/1  "Net Flows (FLOW)"
  Bus Selector/3 -> Product/1  "<Salinity (CONC)>"
  Temperature Balance/1(Out1) -> Bus Creator/1, Scope1/1  "Temperature (T)"
  Bus Selector1/3 -> Product1/2  "<TSD (CONC)>"
  Product/1 -> Salinity Mass Balance/1(InflowLoadingRate1)
  Product1/1 -> Salinity Mass Balance/2(InflowLoadingRate2)
  TSS Mass Balance/1(TSS Concentration (CONC)) -> Scope1/3, Bus Creator/3  "TSS (CONC)"
  Salinity Mass Balance/1(TDS (CONC)) -> Scope1/2, Bus Creator/2  "TDS (CONC)"
  Bus Creator1/1 -> Bus to Vector/1
  Bus to Vector/1 -> MATLAB Function/1(inflows)
  Constant/1 -> MATLAB Function/3(vol), Gain/1, Gain1/1
  Integrator/1 -> MATLAB Function/4(volStored), Scope/1, Temperature Balance/5(Volume), Salinity Mass Balance/5(Volume (L3)), TSS Mass Balance/5(Volume (L3))  "Stored Volume (VOL)"
  Gain/1 -> Scope/3, MATLAB Function/5(upperVol)  "Max Operational Volume (VOL)"
  Gain1/1 -> MATLAB Function/6(lowerVol), Scope/2  "Min Operational Vol (VOL)"
  MATLAB Function/1(newInflows) -> Inflow 1 Flow Rate (FLOW)/1, Inflow 2 Flow Rate (FLOW)/1
  MATLAB Function/4(t) -> Memory/1, Scope2/1  "timer"
  Memory/1 -> Scope2/2, MATLAB Function/7("t ")

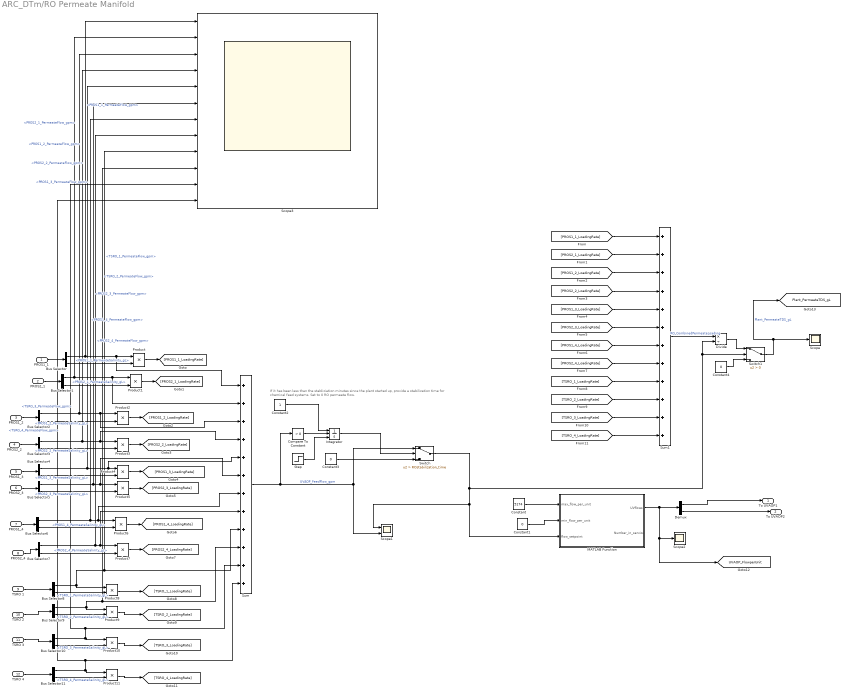
== system ARC_DTm/RO Permeate Manifold ==
  note: If it has been less than the stabliziation minutes since the plant started up, provide a stabilization time for chemical feed systems.
      | Set to 0 RO permeate flow.
  PROS1_1 : Inport
  PROS2_1 : Inport  Port=2
  PROS1_2 : Inport  Port=3
  PROS2_2 : Inport  Port=4
  PROS1_3 : Inport  Port=5
  PROS2_3 : Inport  Port=6
  PROS1_4 : Inport  Port=7
  PROS2_4 : Inport  Port=8
  TSRO 1 : Inport  Port=9
  TSRO 2 : Inport  Port=10
  TSRO 3 : Inport  Port=11
  TSRO 4 : Inport  Port=12
  Bus Selector : BusSelector  OutputSignals=PROS1_1_PermeateFlow_gpm,PROS1_1_PermeateSalinity_gL
  Bus Selector1 : BusSelector  OutputSignals=PROS2_1_PermeateFlow_gpm,PROS2_1_PermeateSalinity_gL
  Bus Selector10 : BusSelector  OutputSignals=TSRO_3_PermeateFlow_gpm,TSRO_3_PermeateSalinity_gL
  Bus Selector11 : BusSelector  OutputSignals=TSRO_4_PermeateFlow_gpm,TSRO_4_PermeateSalinity_gL
  Bus Selector2 : BusSelector  OutputSignals=PROS1_2_PermeateFlow_gpm,PROS1_2_PermeateSalinity_gL
  Bus Selector3 : BusSelector  OutputSignals=PROS2_2_PermeateFlow_gpm,PROS2_2_PermeateSalinity_gL
  Bus Selector4 : BusSelector  OutputSignals=PROS1_3_PermeateFlow_gpm,PROS1_3_PermeateSalinity_gL
  Bus Selector5 : BusSelector  OutputSignals=PROS2_3_PermeateFlow_gpm,PROS2_3_PermeateSalinity_gL
  Bus Selector6 : BusSelector  OutputSignals=PROS1_4_PermeateFlow_gpm,PROS1_4_PermeateSalinity_gL
  Bus Selector7 : BusSelector  OutputSignals=PROS2_4_PermeateFlow_gpm,PROS2_4_PermeateSalinity_gL
  Bus Selector8 : BusSelector  OutputSignals=TSRO_1_PermeateFlow_gpm,TSRO_1_PermeateSalinity_gL
  Bus Selector9 : BusSelector  OutputSignals=TSRO_2_PermeateFlow_gpm,TSRO_2_PermeateSalinity_gL
  Compare To Constant : simulink/Logic and Bit Operations/Compare To Constant  relop=>  const=0  OutDataTypeStr=boolean
  Constant : Constant  Value=5174
  Constant1 : Constant  Value=0
  Constant2 : Constant
  Constant3 : Constant  Value=0
  Constant4 : Constant  Value=0
  Demux : Demux  Outputs=2
  Divide : Product  Inputs=*/
  Integrator : Integrator  ExternalReset=rising  InitialConditionSource=external
  MATLAB Function : MATLAB Function  TreatAsAtomicUnit=on
  Product{,1..11} (12 alike) : Product
  Scope : Scope
      settings: ActiveDisplayYMinimum=-0.0012356397337472099  ActiveDisplayYMaximum=0.011120757603724891  DataLoggingVariableName=ScopeData44
  Scope1 : Scope  NumInputPorts=2
      settings: ActiveDisplayYMinimum=-1294.7457419285424  ActiveDisplayYMaximum=11322.819964623191  DataLoggingVariableName=ScopeData49
  Scope2 : Scope
      settings: ActiveDisplayYMinimum=-646.74999999999989  ActiveDisplayYMaximum=5820.75  DataLoggingVariableName=ScopeData55
  Scope3 : Scope  NumInputPorts=12
      settings: ActiveDisplayYMinimum=-227.64962771948578  ActiveDisplayYMaximum=1886.6487906439902  DataLoggingVariableName=ScopeData63
  Step : Step  Before=ROstabilization_time  After=0  SampleTime=0
  Sum : Sum  Inputs=++++++++++++
  Sum1 : Sum  Inputs=++++++++++++
  Switch : Switch  Criteria=u2 > Threshold  Threshold=ROstabilization_time  SaturateOnIntegerOverflow=off  InputSameDT=off
  Switch1 : Switch  Criteria=u2 > Threshold  SaturateOnIntegerOverflow=off  InputSameDT=off
  To UVAOP1 : Outport
  To UVAOP2 : Outport  Port=2
  tag scope: Plant_PermeateTDS_gL=global, UVAOP_FlowperUnit=global
  wires:
  PROS1_1/1 -> Bus Selector/1
  Bus Selector/2 -> Product/2  "<PROS1_1_PermeateSalinity_gL>"
  Bus Selector/1 -> Scope3/1, Sum/1, Product/1  "<PROS1_1_PermeateFlow_gpm>"
  Product/1 -> [PROS1_1_LoadingRate]
  Bus Selector1/2 -> Product1/2  "<PROS2_1_PermeateSalinity_gL>"
  Bus Selector1/1 -> Scope3/2, Sum/2, Product1/1  "<PROS2_1_PermeateFlow_gpm>"
  Product1/1 -> [PROS2_1_LoadingRate]
  PROS2_1/1 -> Bus Selector1/1
  Bus Selector2/2 -> Product2/2  "<PROS1_2_PermeateSalinity_gL>"
  Bus Selector2/1 -> Scope3/3, Sum/3, Product2/1  "<PROS1_2_PermeateFlow_gpm>"
  Product2/1 -> [PROS1_2_LoadingRate]
  PROS1_2/1 -> Bus Selector2/1
  Bus Selector3/2 -> Product3/2  "<PROS2_2_PermeateSalinity_gL>"
  Bus Selector3/1 -> Scope3/4, Sum/4, Product3/1  "<PROS2_2_PermeateFlow_gpm>"
  Product3/1 -> [PROS2_2_LoadingRate]
  PROS2_2/1 -> Bus Selector3/1
  Bus Selector4/2 -> Product4/2  "<PROS1_3_PermeateSalinity_gL>"
  Bus Selector4/1 -> Scope3/5, Sum/5, Product4/1  "<PROS1_3_PermeateFlow_gpm>"
  Product4/1 -> [PROS1_3_LoadingRate]
  PROS1_3/1 -> Bus Selector4/1
  Product5/1 -> [PROS2_3_LoadingRate]
  PROS2_3/1 -> Bus Selector5/1
  Bus Selector5/1 -> Scope3/6, Sum/6, Product5/1  "<PROS2_3_PermeateFlow_gpm>"
  Bus Selector5/2 -> Product5/2  "<PROS2_3_PermeateSalinity_gL>"
  Bus Selector6/1 -> Scope3/7, Sum/7, Product6/1  "<PROS1_4_PermeateFlow_gpm>"
  Product6/1 -> [PROS1_4_LoadingRate]
  Bus Selector6/2 -> Product6/2  "<PROS1_4_PermeateSalinity_gL>"
  Bus Selector7/1 -> Scope3/8, Sum/8, Product7/1  "<PROS2_4_PermeateFlow_gpm>"
  Product7/1 -> [PROS2_4_LoadingRate]
  PROS2_4/1 -> Bus Selector7/1
  Bus Selector7/2 -> Product7/2  "<PROS2_4_PermeateSalinity_gL>"
  PROS1_4/1 -> Bus Selector6/1
  [PROS1_1_LoadingRate] -> Sum1/1
  [PROS2_1_LoadingRate] -> Sum1/2
  [PROS1_2_LoadingRate] -> Sum1/3
  [PROS2_2_LoadingRate] -> Sum1/4
  [PROS1_4_LoadingRate] -> Sum1/7
  [PROS2_4_LoadingRate] -> Sum1/8
  [PROS2_3_LoadingRate] -> Sum1/6
  [PROS1_3_LoadingRate] -> Sum1/5
  [TSRO_3_LoadingRate] -> Sum1/11
  [TSRO_2_LoadingRate] -> Sum1/10
  [TSRO_1_LoadingRate] -> Sum1/9
  TSRO 1/1 -> Bus Selector8/1
  Bus Selector8/1 -> Scope3/9, Sum/9, Product8/1  "<TSRO_1_PermeateFlow_gpm>"
  Bus Selector8/2 -> Product8/2  "<TSRO_1_PermeateSalinity_gL>"
  Product8/1 -> [TSRO_1_LoadingRate]
  Bus Selector9/1 -> Product9/1, Scope3/10, Sum/10  "<TSRO_2_PermeateFlow_gpm>"
  Product9/1 -> [TSRO_2_LoadingRate]
  Bus Selector9/2 -> Product9/2  "<TSRO_2_PermeateSalinity_gL>"
  TSRO 2/1 -> Bus Selector9/1
  Bus Selector10/1 -> Sum/11, Scope3/11, Product10/1  "<TSRO_3_PermeateFlow_gpm>"
  Product10/1 -> [TSRO_3_LoadingRate]
  Bus Selector10/2 -> Product10/2  "<TSRO_3_PermeateSalinity_gL>"
  TSRO 3/1 -> Bus Selector10/1
  Bus Selector11/1 -> Sum/12, Scope3/12, Product11/1  "<TSRO_4_PermeateFlow_gpm>"
  Product11/1 -> [TSRO_4_LoadingRate]
  Bus Selector11/2 -> Product11/2  "<TSRO_4_PermeateSalinity_gL>"
  TSRO 4/1 -> Bus Selector11/1
  Sum1/1 -> Divide/1  "RO_CombinedPermeateLoading"
  Switch1/1 -> [Plant_PermeateTDS_gL], Scope/1  "Plant_PermeateTDS_gL"
  MATLAB Function/1(UVflows) -> Scope2/1, [UVAOP_FlowperUnit], Demux/1
  Demux/1 -> To UVAOP1/1
  Demux/2 -> To UVAOP2/1
  Constant/1 -> MATLAB Function/1(max_flow_per_unit)
  Constant1/1 -> MATLAB Function/2(min_flow_per_unit)
  Constant3/1 -> Switch/3
  Integrator/1 -> Switch/2
  Sum/1 -> Switch/1, Scope1/2, Compare To Constant/1  "UVAOP_FeedFlow_gpm"
  Compare To Constant/1 -> Integrator/2
  Constant2/1 -> Integrator/1
  Switch/1 -> Switch1/2, Divide/2, Scope1/1, MATLAB Function/3(flow_setpoint)
  Step/1 -> Integrator/3
  [TSRO_4_LoadingRate] -> Sum1/12
  Divide/1 -> Switch1/1
  Constant4/1 -> Switch1/3

== system ARC_DTm/Subsystem1 ==
  Add : Sum  Inputs=++++
  Bus Creator : BusCreator  Inputs=21
  Demux : Demux
  Demux1 : Demux
  Demux2 : Demux  Outputs=2
  Demux3 : Demux
  Display : Display
  GPM>MGm : Gain  Gain=1/1000000
  Integrator : Integrator
  Scope : Scope  NumInputPorts=4
      settings: ActiveDisplayYMinimum=-337.49999999999994  ActiveDisplayYMaximum=3037.5  DataLoggingVariableName=ScopeData7
  Scope1 : Scope  NumInputPorts=2
      settings: ActiveDisplayYMinimum=-8.659250749740238  ActiveDisplayYMaximum=77.933256747662156  DataLoggingVariableName=ScopeData9
  Scope3 : Scope
      settings: ActiveDisplayYMinimum=-0.0012576329242460021  ActiveDisplayYMaximum=0.011318696318214021  DataLoggingVariableName=ScopeData54
  Scope4 : Scope  NumInputPorts=2
      settings: ActiveDisplayYMinimum=-646.74999999999989  ActiveDisplayYMaximum=5820.75  DataLoggingVariableName=ScopeData59
  Sum : Sum  Inputs=|++
  To Workspace : ToWorkspace  VariableName=flows  SaveFormat=Timeseries  SampleTime=-1
  Total Permeate Production : Integrator
  gal > MG : Gain  Gain=1/1000000
  wires:
  [PRO_FlowperUnit_gpm] -> Demux/1, Scope/1  "PRO Flows"
  [TSRO_UnitFlows] -> Demux1/1, Scope/2  "TSRO Flows"
  [UVAOP_FlowperUnit] -> Demux2/1, Scope/3
  [UFPump_FlowperUnit] -> Scope/4, Demux3/1
  Demux/1 -> Bus Creator/4  "PRO_1_FeedFlow_gpm"
  Demux/2 -> Bus Creator/5  "PRO_2_FeedFlow_gpm"
  Demux/3 -> Bus Creator/6  "PRO_3_FeedFlow_gpm"
  Demux/4 -> Bus Creator/7  "PRO_4_FeedFlow_gpm"
  Demux1/1 -> Bus Creator/8  "TSRO_1_FeedFlow_gpm"
  Demux1/2 -> Bus Creator/9  "TSRO_2_FeedFlow_gpm"
  Demux1/3 -> Bus Creator/10  "TSRO_3_FeedFlow_gpm"
  Demux1/4 -> Bus Creator/11  "TSRO_4_FeedFlow_gpm"
  Demux2/1 -> Bus Creator/12, Scope4/1, Sum/1  "UVAOP_1_FeedFlow_gpm"
  Demux2/2 -> Scope4/2, Bus Creator/13, Sum/2  "UVAOP_2_FeedFlow_gpm"
  Sum/1 -> Bus Creator/2, GPM>MGm/1  "Plant_PermeateProduction_gpm"
  Demux3/1 -> Bus Creator/14, Add/1  "UFPump_1_FeedFlow_gpm"
  Demux3/2 -> Bus Creator/15, Add/2  "UFPump_2_FeedFlow_gpm"
  Demux3/3 -> Bus Creator/16, Add/3  "UFPump_3_FeedFlow_gpm"
  Demux3/4 -> Bus Creator/17, Add/4  "UFPump_4_FeedFlow_gpm"
  Add/1 -> Bus Creator/3  "Plant_FeedFlow_gpm"
  GPM>MGm/1 -> Scope3/1, Total Permeate Production/1
  Total Permeate Production/1 -> Scope1/1, Display/1, Bus Creator/1  "Plant_TotalPermeateProduction_MG"
  Bus Creator/1 -> To Workspace/1
  [Plant_BrineOut] -> gal > MG/1, Bus Creator/18  "Plant_BrineFlow_gpm"
  gal > MG/1 -> Integrator/1  "Plant_TotalBrineProduction_MG"
  Integrator/1 -> Bus Creator/19, Scope1/2  "Plant_TotalBrineProduction_MG"
  [Plant_PermeateTDS_gL] -> Bus Creator/20  "Plant_PermeateTDS_gL"
  [Plant_BrineTDS_gL] -> Bus Creator/21  "Plant_BrineTDS_gL"

== system ARC_DTm/TSRO Concentrate Manifold ==
  TSRO1_Concentrate : Inport
  TSRO2_Concentrate : Inport  Port=2
  TSRO3_Concentrate : Inport  Port=3
  TSRO4_Concentrate : Inport  Port=4
  Bus Selector : BusSelector  OutputSignals=TSRO_1_BrineFlow_gpm,TSRO_1_BrineConductivity_gL,TSRO_1_ConcentratePressure_psi
  Bus Selector1 : BusSelector  OutputSignals=TSRO_2_BrineFlow_gpm,TSRO_2_BrineConductivity_gL,TSRO_2_ConcentratePressure_psi
  Bus Selector2 : BusSelector  OutputSignals=TSRO_3_BrineFlow_gpm,TSRO_3_BrineConductivity_gL,TSRO_3_ConcentratePressure_psi
  Bus Selector3 : BusSelector  OutputSignals=TSRO_4_BrineFlow_gpm,TSRO_4_BrineConductivity_gL,TSRO_4_ConcentratePressure_psi
  Constant : Constant  Value=0
  Product : Product  Inputs=*/
  Scope : Scope  NumInputPorts=2
      settings: ActiveDisplayYMinimum=3.0176317562217632  ActiveDisplayYMaximum=8.0162337431516359  DataLoggingVariableName=ScopeData22
  Switch : Switch  Criteria=u2 > Threshold  SaturateOnIntegerOverflow=off  InputSameDT=off
  TSRO1_LoadingRate : Product
  TSRO2_LoadingRate : Product
  TSRO3_LoadingRate : Product
  TSRO4_LoadingRate : Product
  TSRO_BrineFlow : Scope
      settings: ActiveDisplayYMinimum=-1  ActiveDisplayYMaximum=1  DataLoggingVariableName=ScopeData15
  TSRO_TotalConcFlow_gpm : Sum  Inputs=++++
  TSRO_TotalConcLoading : Sum  Inputs=++++
  tag scope: Plant_BrineOut=global, Plant_BrineTDS_gL=global
  wires:
  TSRO1_Concentrate/1 -> Bus Selector/1
  TSRO2_Concentrate/1 -> Bus Selector1/1
  TSRO4_Concentrate/1 -> Bus Selector3/1
  TSRO3_Concentrate/1 -> Bus Selector2/1
  Bus Selector/1 -> TSRO1_LoadingRate/1, TSRO_TotalConcFlow_gpm/1  "<TSRO_1_BrineFlow_gpm>"
  Bus Selector/2 -> TSRO1_LoadingRate/2  "<TSRO_1_BrineConductivity_gL>"
  Bus Selector2/1 -> TSRO3_LoadingRate/1, TSRO_TotalConcFlow_gpm/2  "<TSRO_3_BrineFlow_gpm>"
  Bus Selector2/2 -> TSRO3_LoadingRate/2  "<TSRO_3_BrineConductivity_gL>"
  Bus Selector3/2 -> TSRO4_LoadingRate/2  "<TSRO_4_BrineConductivity_gL>"
  Bus Selector3/1 -> TSRO_TotalConcFlow_gpm/3, TSRO4_LoadingRate/1  "<TSRO_4_BrineFlow_gpm>"
  Bus Selector1/1 -> TSRO_TotalConcFlow_gpm/4, TSRO2_LoadingRate/1  "<TSRO_2_BrineFlow_gpm>"
  Bus Selector1/2 -> TSRO2_LoadingRate/2  "<TSRO_2_BrineConductivity_gL>"
  TSRO1_LoadingRate/1 -> TSRO_TotalConcLoading/1
  TSRO3_LoadingRate/1 -> TSRO_TotalConcLoading/2
  TSRO4_LoadingRate/1 -> TSRO_TotalConcLoading/3
  TSRO2_LoadingRate/1 -> TSRO_TotalConcLoading/4
  TSRO_TotalConcFlow_gpm/1 -> TSRO_BrineFlow/1, Switch/2, Product/2, [Plant_BrineOut]
  TSRO_TotalConcLoading/1 -> Product/1
  Product/1 -> Switch/1, Scope/1
  Constant/1 -> Switch/3
  Switch/1 -> [Plant_BrineTDS_gL], Scope/2

== system ARC_DTm/TSRO_1 ==
  note: Units needed:
      | u = cm/sec
      | dh = cm
      | Concentrations = g/L
      | Jw_prev = L/m2/min
      |  = Q (Lpm) / Atot(m2)
      | T = oC
      | q = cm/sec =
      | Q (m3/sec) / Atot (m2)
  Inflow : Inport
  Brine Check Valve : Saturate  UpperLimit=Inf  LowerLimit=0
  Brine Flow (gpm) : Sum  Inputs=-+
  Bus Creator : BusCreator  Inputs=2
  Bus Creator1 : BusCreator  Inputs=3
  Bus Selector : BusSelector  OutputSignals=TSRO Feed Pressure _Bar,Feed Temperature (oC),TSRO_FeedTDS_gL,TSRO_1_FeedFlow_gpm
  Bus Selector1 : BusSelector  OutputSignals=TSRO_A,TSRO_B,TSRO_Area_m2
  Channel Area (m2) : Product  Inputs=4
  Check Valve : Saturate  UpperLimit=Inf  LowerLimit=0
  Elements per Vessel : Constant  Value=7
  Feed Channel Height (m) : Constant  Value=L
  Fouling Factor : Constant  Value=1-FF
  Gain : Gain  Gain=3.785
  Initial units : Gain  Gain=10^-8
  Jw_Previous : Memory  InitialCondition=.03
  "L -> gal" : Gain  Gain=1/3.785
  L>m3 : Gain  Gain=1/1000
  MATLAB Function1 : MATLAB Function  TreatAsAtomicUnit=on
  MATLAB Function2 : MATLAB Function  TreatAsAtomicUnit=on
  Membrane Width (m) : Constant  Value=w
  Min : MinMax  Inputs=2
  Minus : Sum  Inputs=+-|
  Number of Vessels : Constant  Value=15
  Pa > Bar : Gain  Gain=100000
  Permeate Flow (gpm) : Product
  Product : Product  Inputs=*/
  Product2 : Product
  Q (L/min) : Gain  Gain=3.785
  Scope : Scope
      settings: ActiveDisplayYMinimum=-1  ActiveDisplayYMaximum=1  DataLoggingVariableName=ScopeData76
  Scope1 : Scope
      settings: ActiveDisplayYMinimum=-188.84815571077934  ActiveDisplayYMaximum=426.44465787754609  DataLoggingVariableName=ScopeData31
  Scope2 : Scope
      settings: ActiveDisplayYMinimum=-95.921175791719065  ActiveDisplayYMaximum=315.81911958419477  DataLoggingVariableName=ScopeData32
  Scope3 : Scope  NumInputPorts=3
      settings: ActiveDisplayYMinimum=-153.08463833077985  ActiveDisplayYMaximum=609.80940425897552  DataLoggingVariableName=ScopeData17
  Spacer Thickness (mm) : Constant  Value=h
  Subsystem : Subsystem
  bar>psi : Gain  Gain=1/.069
  cperm_previous : Memory  InitialCondition=.008
  gpm > L : Gain  Gain=3.785
  initial Units : Gain  Gain=10^-11
  m/min > cm/sec : Gain  Gain=100/60
  m3 > L : Gain  Gain=1000
  m3 > L1 : Gain  Gain=1000
  m>cm : Gain  Gain=100
  m>mm : Gain  Gain=1000
  mm>  cm : Gain  Gain=.1
  mm>m : Gain  Gain=.001
  psi to Bar : Gain  Gain=.069
  s > min : Gain  Gain=60
  s > min1 : Gain  Gain=60
  TSRO_Permeate : Outport
  TSRO_Brine : Outport  Port=2
  tag scope: TSRO_1_deltaPi=global
  wires:
  m/min > cm/sec/1 -> Subsystem/11(u)
  [TSRO_MembraneConstants] -> Bus Selector1/1
  m3 > L1/1 -> s > min1/1
  Bus Selector/1 -> Min/1, Scope/1, bar>psi/1, Subsystem/2(<S2 Feed Pressure (bar)>)  "<TSRO Feed Pressure _Bar>"
  Bus Selector1/3 -> Permeate Flow (gpm)/2  "<TSRO_Area_m2>"
  Membrane Width (m)/1 -> Channel Area (m2)/1, m>mm/1
  [RO_PermeatePressure] -> psi to Bar/1  "Permeate Pressure (psi)"
  Inflow/1 -> Bus Selector/1
  Bus Selector1/1 -> initial Units/1  "<TSRO_A>"
  Bus Selector1/2 -> Initial units/1  "<TSRO_B>"
  Permeate Flow (gpm)/1 -> Check Valve/1  "TSRO_1_PermeateFlow_gpm"
  Bus Selector/2 -> Subsystem/1(<Feed Temperature (oC)>)  "<Feed Temperature (oC)>"
  Bus Selector/3 -> MATLAB Function2/5(cfeed), Subsystem/6(<S2 Feed Salinity (g/L)>)  "<TSRO_FeedTDS_gL>"
  Bus Selector/4 -> Scope3/3, Brine Flow (gpm)/2, Q (L/min)/1  "<TSRO_1_FeedFlow_gpm>"
  Product/1 -> m/min > cm/sec/1
  psi to Bar/1 -> Min/2  "Pressure (bar)"
  MATLAB Function2/1(cbrine) -> Bus Creator1/2  "TSRO_1_BrineConductivity_gL"
  initial Units/1 -> m3 > L/1
  Initial units/1 -> m3 > L1/1
  Spacer Thickness (mm)/1 -> MATLAB Function1/2(h), mm>m/1
  m3 > L/1 -> s > min/1
  Min/1 -> Subsystem/3(Pperm)
  mm>m/1 -> Channel Area (m2)/2
  Channel Area (m2)/1 -> Product/2
  Q (L/min)/1 -> MATLAB Function2/4(Qfeed), L>m3/1  "Qtot (L/min)"
  Bus Creator/1 -> Scope2/1, TSRO_Permeate/1  "TSRO_1_PermeateFlow"
  Number of Vessels/1 -> Channel Area (m2)/3
  s > min/1 -> Pa > Bar/1
  Elements per Vessel/1 -> Channel Area (m2)/4
  s > min1/1 -> Subsystem/5(Salt Perm (L/m2/min))  "Salt Perm (L/m2/min)"
  Fouling Factor/1 -> Product2/2
  m>mm/1 -> MATLAB Function1/1(W)
  L>m3/1 -> Product/1
  Pa > Bar/1 -> Product2/1  "Water Perm (L/m2/min/Bar)"
  MATLAB Function1/1(dh) -> mm>  cm/1
  Feed Channel Height (m)/1 -> m>cm/1
  Jw_Previous/1 -> Subsystem/8(Jw)  "Jw"
  cperm_previous/1 -> Subsystem/7(cperm)  "cperm"
  m>cm/1 -> Subsystem/10(L)
  Product2/1 -> Subsystem/4(Water Perm (L/m2/min/Bar))  "Water Perm (L/m2/min/Bar)"
  Gain/1 -> MATLAB Function2/2(Qperm)  "Predicted Permeate Flow (L/min)"
  mm>  cm/1 -> Subsystem/9(dh)
  Bus Creator1/1 -> Scope1/1, TSRO_Brine/1  "TSRO_Feedwater"
  bar>psi/1 -> Minus/1  "TSRO_1_ConcentratePressure_psi"
  Subsystem/1(Permeate Flux Rate (L/min/m2)) -> Jw_Previous/1, "L -> gal"/1  "Permeate Flux Rate* (L/min.m2)"
  Subsystem/2(Permeate Salinity g/L) -> Bus Creator/2, MATLAB Function2/1(cperm), cperm_previous/1  "TSRO_1_PermeateSalinity_gL"
  "L -> gal"/1 -> Permeate Flow (gpm)/1
  Subsystem/3(deltaPi_bar) -> [TSRO_1_deltaPi]
  Brine Check Valve/1 -> gpm > L/1, Scope3/2, Bus Creator1/1  "TSRO_1_BrineFlow_gpm"
  gpm > L/1 -> MATLAB Function2/3(Qbrine)
  [TSRO_Suction_PressureDrop_psi] -> Minus/2
  Minus/1 -> Bus Creator1/3  "TSRO_1_ConcentratePressure_psi"
  Brine Flow (gpm)/1 -> Brine Check Valve/1  "TSRO_1_BrineFlow_gpm"
  Check Valve/1 -> Brine Flow (gpm)/1, Scope3/1, Bus Creator/1, Gain/1  "TSRO_1_PermeateFlow_gpm"
